simulink subsystem "Nonlinear_model"  (R2021b)
settings: Solver=VariableStepAuto  StartTime=0.0  StopTime=10.0  RelTol=1e-3
undefined symbols (not defined in the file): Q1, Q2, R
libraries: simulink x2
settings Model: Creator=aakas  LastModifiedBy=aakas

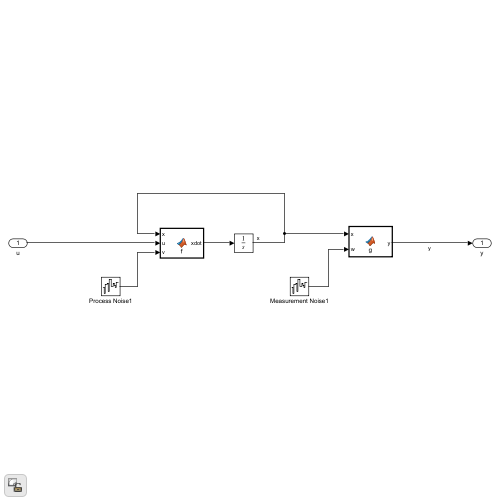
[thumbnail: Simulink's stored preview of the top-level diagram]
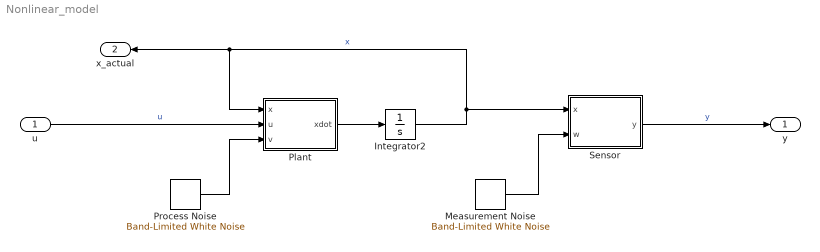
== system Nonlinear_model ==
  u : Inport
  Integrator2 : Integrator  InitialCondition=[0; 0]
  Measurement Noise : simulink/Sources/Band-Limited White Noise  Cov=R*0.1  Ts=0.1  seed=[32523]
  Plant : MATLAB Function  TreatAsAtomicUnit=on
  Process Noise : simulink/Sources/Band-Limited White Noise  Cov=[Q1; Q2]*0.1  Ts=0.1  seed=[23341]
  Sensor : MATLAB Function  TreatAsAtomicUnit=on
  y : Outport
  x_actual : Outport  Port=2
  wires:
  u/1 -> Plant/2(u)  "u"
  Integrator2/1 -> Sensor/1(x), Plant/1(x), x_actual/1  "x"
  Plant/1(xdot) -> Integrator2/1
  Measurement Noise/1 -> Sensor/2(w)
  Process Noise/1 -> Plant/3(v)
  Sensor/1(y) -> y/1  "y"

== matlab function Nonlinear_model/Plant ==
  data: x input; u input; xdot output; v input
function xdot = f(x,u,v)

xdot = [x(2); (1-x(1)^2)*x(2)-x(1)] + v;

== matlab function Nonlinear_model/Sensor ==
  data: x input; w input; y output
function y = g(x,w)

y = x*(1+w);
